simulink model "aufgabe22simulink"  (R2014a)
settings: Solver=ode45  StartTime=0.0  StopTime=10.0  RelTol=1e-3
values from neighbouring files (symbols this model uses):
  C = T/R    (= 0.01)    [Aufgabe22.m]
  R = 1e3    (= 1000)    [Aufgabe22.m]
settings Model: Creator=s55812  LastModifiedBy=s55812

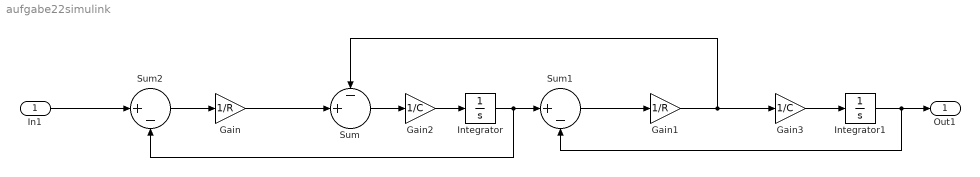
== system aufgabe22simulink ==
  In1 : Inport
  Gain : Gain  Gain=1/R
  Gain1 : Gain  Gain=1/R
  Gain2 : Gain  Gain=1/C
  Gain3 : Gain  Gain=1/C
  Integrator : Integrator
  Integrator1 : Integrator
  Sum : Sum  Inputs=-+|
  Sum1 : Sum  Inputs=|+-
  Sum2 : Sum  Inputs=|+-
  Out1 : Outport
  wires:
  Gain/1 -> Sum/2
  Sum1/1 -> Gain1/1
  Sum2/1 -> Gain/1
  Gain1/1 -> Sum/1, Gain3/1
  Sum/1 -> Gain2/1
  In1/1 -> Sum2/1
  Integrator/1 -> Sum2/2, Sum1/1
  Integrator1/1 -> Sum1/2, Out1/1
  Gain3/1 -> Integrator1/1
  Gain2/1 -> Integrator/1
